simulink model "stackedRotor_dualEMRAX_dynInflow"  (R2022b)
settings: Solver=ode45  StartTime=0.0  StopTime=60  RelTol=1e-4  EnableMultiTasking=on
InitFcn:
  | %Hide scope plots
  | HidHandles = get(0,'ShowHiddenHandles');
  | set(0,'ShowHiddenHandles','On');
  | AllScopeHandles = findobj(0,'Type','Figure','Tag','SIMULINK_SIMSCOPE_FIGURE');
  | close(AllScopeHandles);
  | set(0,'ShowHiddenHandles',HidHandles);
  | 
  | %Load Cl and Cd from potential flow
  | load('C:\Users\msa2925\Box\Matt Lab Stuff\5th Year\Modeling\Look Up Tables\ClCd-1.mat');
  | 
  | %Load dynamic inflow properties (model and rotor_params)
  | load('C:\Users\msa2925\Box\Matt Lab Stuff\5th Year\Modeling\Look Up Tables\DynInflow-1.mat');
  | 
  | 
  | %Atmospheric Properties
  | rho_air    = 1.225;  % air density in kg/m^3
  | mu         = 1.803e-5; % dynamic viscosity [N-s/m^2]
  | 
  | %Emrax 208 Electrical Properties
  | R          = .0122;  %  resistance, ohms, line-line at room temp
  | L          = 125*10^-6;  %  inductance line-line at commutation frequency, henries
  | t_elec     = L/R;
  | Imotor     = 256/100^2;  %  kg*m^2 -- From Emrax data sheet
  | Kt_motor   = .80;  %  N*m/Arms
  | Ke_motor   = .0487*sqrt(2)*60/(2*pi);  %  Vpk/rad/sec
  | Ke         = .0487*sqrt(2)*60/(2*pi);   %radians/sec
  | POLES      = 20;
  | 
  | % no-load current fit (i0 = a1*omega^2 + a2) [Apk]
  | i_a1 = 8.98e-5;
  | i_a2 = 2.51;
  | 
  | %-----------Controller Properties------------------%
  | Vbus                 = 175;  % Actual bus voltage (volts) that will be applied
  | CurrentSenseMax      = 250;  %  Max current sense from controller code
  | BASE_CURRENT         = 125;   %  Max current in amps corresponding to normalized control loop current = 1
  | LOOP_FREQUENCY       = 35;     % orig: 35 in kHz
  | T_LOOP               = .001/LOOP_FREQUENCY;
  | pwm_loop_prescalar   = 1;  %Presacalar how many PWM cycles for one current loop execution
  | T_PWM                = T_LOOP/pwm_loop_prescalar;  %  Current loop prescaler on PWM is 1 for Uber
  | BASE_FREQ            = 1200; %POLES/2*1300/60;  %  1300 rpm
  | BaseSpeed            = BASE_FREQ*(60.0/(POLES/2.0));
  | omega                = 0;               % omega for de-coupling integrator
  | MsgFreq              = 1000; %Hz
  | 
  | %Current loop
  | alpha    = 250*2*pi;         % current loop bandwidth
  | I_Kp     = alpha*L*1;
  | I_Ki     = alpha*R/I_Kp*T_LOOP;
  | 
  | %Speed loop
  | SpeedLoopPrescale  = 5;
  | Tspeedloop         = T_LOOP*SpeedLoopPrescale;
  | PID_spd_Kp         = 4.75;   % From Uber code (ORIGINIAL: 3)
  | % PID_spd_Ki         = 2.1*Tspeedloop*1.5;   % From Uber code (ORIGINAL: 0.15*Tspeedloop*2)
  | PID_spd_Ki         = 1.75*Tspeedloop;
  | 
  | %Position loop
  | speedErrorPEngage    = .003; % Speed error max for position loop to enable
  | % Code has .001 for PEngage, trying something diff here
  | PID_pos_Kp           = 4.75; %on MC40: 2.5 (changed on 23 OCT 2021 to 3.5)
  | PID_pos_Ki           = 1e-3; % orig: 0.00003. increase for faster response.
  | PID_pos_Kd           = 8000; % on MC40: 8000.
  | 
  | PID_pos_error_sat   = .3;  % ORIG = 0.3 Maximum error saturated into position PID (in simulink, not C right now)
  | PID_pos_sat         = 1;  %  From code, based on DC bus limit (orig: .25)
  | PID_pos_C1          = .999; % ORIG = 1 Position loop D bandlimit filter
  | PID_pos_C2          = .001;  % ORIG = 0 Position loop D bandlimit filter
  | 
  | 
  | %transfer function of speed estimator is K1*K3*z/(z-K2)
  | %  Pole is at z = K2
  | % z = exp(-sT)
  | f_estpole = 35000;  %orig: 35000
  | K1        = 1/(BASE_FREQ*T_LOOP);   %  Divide by base freq to convert from elec delta-normalized-angle/cycle to [0,1] normalized speed
  |                                     %  K1 converts delta angle estimate over a loop period to a [0,1] speed estimate
  | K2        = exp(-f_estpole*2*pi*T_LOOP);
  | K3        = 1 - K2;  % Set to make filter have unity gain at 0 frequency (z = 1)
  | 
  | %----------------Rotor properties----------------%
  | d_prop      = 2.216;   %  diameter propeller [m] 2.032 (coax) 2.216 (uber)
  | c           = 0.08; %chord [m]
  | nb          = 2; %number of blades
  | sigma       = nb*c/pi/(d_prop/2);
  | GR          = 1; %gear ratio
  | %Iload        = 0.3578*(1/GR)^2; (coax rotor inertia)
  | %inertias (stacked) measured from 230929 and 231003 testing
  | Im_upper    = 0.3662; %kg-m2
  | Im_lower    = 0.3540;
  | Ir_upper    = 0.3124;
  | Ir_lower    = 0.3317;
  | 
  | %from stacked dual motor testing, coax hubs (220403_test_b)
  | %Iload       = 0.3578/2*(1/GR)^2; %from stacked dual motor testing (231023_test_b)
  | % Iload       = I_eff + Idrive + Imotor;
  | 
  | 
  | %------------Inputs---------------%
  | Ang_slew       = 15.83; % deg/s
  | Ramp_sec       = 100; % rpm/s
  | InitialRPM     = 950*GR;
  | omegamech      = InitialRPM/60*2*pi;  %  Used to preload Q current voltage integrator
  | t_ang_step     = 2; %timestep for angle commands
  | t_swept        = 10; %time to send swept sine input
values from neighbouring files (symbols this model uses):
  AoA_sweep = [-2 -1 0 1 2 3 4 5 6 7 8 9 ... (13 elements, 1x13)]    [ClCd-1.mat]
  Cdl = [0.0123 0.0123 0.0123 0.0123 0.0123 0.0123 0.0123 0.0123 0.0123 0.0123 0.0123 0.0123 ... (6500 elements, 13x500)]    [ClCd-1.mat]
  Cdu = [0.0123 0.0123 0.0123 0.0123 0.0123 0.0123 0.0123 0.0123 0.0123 0.0123 0.0123 0.0123 ... (6500 elements, 13x500)]    [ClCd-1.mat]
  Cll = [-0.111113403346 0.00796289645531 0.127036770682 0.246071948277 0.365032169973 0.483881199334 0.602582833794 0.721100915686 0.839399343253 0.957442081649 1.07519317391 1.19261675192 ... (6500 elements, 13x500)]    [ClCd-1.mat]
  Clu = [-0.11705321178 0.00839337636768 0.133837407812 0.259240671085 0.384564967138 0.509772120977 0.634823993289 0.759682492064 0.884309584192 1.00866730705 1.13271778008 1.2564232163 ... (6500 elements, 13x500)]    [ClCd-1.mat]
  Cp = [0.000195201118563 0.000195344815163 0.000195970524669 0.000196911243155 0.000198292722473 0.000199793715635 0.000201836164013 0.000204359459521 0.00020706119236 0.00020992934584 0.000212955219574 0.000216131124695 ... (150 elements, 1x150)]    [BEMT-1.mat]    (also in BEMT-2.mat = [5.908e-05 5.908e-05 5.908e-05 5.908e-05 5.908e-05 5.908e-05; BEMT-3.mat = [6.167e-05 6.167e-05 6.167e-05 6.167e-05 6.167e-05 6.1671725; BEMT-PF-Isolated-1.mat = [6.88284627296e-05 6.76929537705e-05 6.92283244838e-05 7.518; BEMT-PF-Isolated-2.mat = [6.88286203447e-05 6.76929720507e-05 6.92293837373e-05 7.518)
  Cpl = [0.000333700998998 0.000390181039031 0.000394788670278 0.000400729506228 0.000408611755119 0.000419410254194 0.000434611180529 0.000454621522012 0.000471293145772 0.000468819202162 0.000461044856051 0.0004465872684 ... (37 elements, 1x37)]    [BEMT-PF-Stacked-1.mat]    (also in BEMT-PF-Stacked-3.mat = [0.00012095698162 0.000162284223538 0.000164817714818 0.0001; BEMT-PF-Stacked-4.mat = [0.000215313097577 0.00022323140747 0.000225181363314 0.0002; BEMT-PF-Stacked-5.mat = [0.000201399004141 0.000209364989981 0.000211223578331 0.000; CpData-Stacked-1.mat = [0.0004204989393 0.000429722690454 0.000432518606247 0.00043)
  Cpu = [0.000372640330495 0.000318761476241 0.00031503993434 0.000310316169544 0.000304143730405 0.000295773643033 0.00028387117424 0.000265492168428 0.000237641915024 0.000230728320611 0.000223594040333 0.000216887343718 ... (37 elements, 1x37)]    [BEMT-PF-Stacked-1.mat]    (also in BEMT-PF-Stacked-3.mat = [0.00014995136179 0.000108984048023 0.00010569458686 0.00010; BEMT-PF-Stacked-4.mat = [0.000200079302516 0.0001931098957 0.000191441123461 0.00018; BEMT-PF-Stacked-5.mat = [0.000223261524278 0.000214635121691 0.000212581398187 0.000; CpData-Stacked-1.mat = [0.000470292570894 0.000463315827435 0.000462372188797 0.000)
  Ct = [0 8.42066058624e-05 0.000168413211725 0.000252619817587 0.000348569118235 0.000435711397794 0.000522853677352 0.000609995956911 0.00069713823647 0.000784280516029 0.000871422795587 0.000958565075146 ... (150 elements, 1x150)]    [BEMT-1.mat]    (also in BEMT-2.mat = [-0.000241284312952 -0.00019885713846 -0.000156429963968 -0.; BEMT-3.mat = [-0.000252881464423 -0.00020500571035 -0.00015767832519 -0.0; BEMT-PF-Isolated-1.mat = [-0.000124730397385 6.78902114512e-07 0.000152796242494 0.00; BEMT-PF-Isolated-2.mat = [-0.000124743531158 6.68801957239e-07 0.000152879013625 0.00)
  Ctl = [0.00438668608339 0.0050628698524 0.00511522584539 0.00518172746808 0.00526807639226 0.00538256546486 0.00553531477508 0.00571551109899 0.00580582681419 0.00575766596858 0.00565748394784 0.00549586936617 ... (37 elements, 1x37)]    [BEMT-PF-Stacked-1.mat]    (also in BEMT-PF-Stacked-2.mat = [0.00446656952376 0.00504151525843 0.00508284852112 0.005134; BEMT-PF-Stacked-3.mat = [0.00184996435909 0.00209589101081 0.00210506301257 0.002127; BEMT-PF-Stacked-4.mat = [0.00305779502317 0.00317485141984 0.00320289061972 0.003237; BEMT-PF-Stacked-5.mat = [0.00284078729023 0.00295761000687 0.00298453442892 0.003017)
  Ctu = [0.00485875244254 0.00420098979139 0.00415434112966 0.00409491081367 0.00401692201007 0.00391066006909 0.00375881977479 0.00352379292731 0.0031675839941 0.00307949239151 0.00298865074931 0.00290335167779 ... (37 elements, 1x37)]    [BEMT-PF-Stacked-1.mat]    (also in BEMT-PF-Stacked-2.mat = [0.00487929290239 0.00430977798758 0.00426987840094 0.004219; BEMT-PF-Stacked-3.mat = [0.00202552929257 0.00178155832272 0.00175724958711 0.001735; BEMT-PF-Stacked-4.mat = [0.00282403441036 0.00271496837402 0.00268870985611 0.002655; BEMT-PF-Stacked-5.mat = [0.00315608603824 0.00303364263049 0.00300412792098 0.002966)
  index_sweep = [-90 -45 -40 -35 -30 -25 -20 -15 -10 -9 -8 -7 ... (37 elements, 1x37)]    [BEMT-PF-Stacked-1.mat]    (also in BEMT-PF-Stacked-2.mat; BEMT-PF-Stacked-3.mat = [-90 -45 -40 -35 -30 -25 -20 -15 -14 -13 -12 -11 ... (45 ele; BEMT-PF-Stacked-4.mat; BEMT-PF-Stacked-5.mat)
  index_sweep_Cp_table = [-90 -45.2679945682 -41.0748847617 -35.9788199136 -30.8261561384 -25.6873115637 -20.5477936424 -15.3629851439 -10.3005197032 -7.23856497031 -5.29357093665 -4.47027434572 ... (27 elements, 1x27)]    [CpData-Stacked-1.mat]
  model =     [DynInflow-1.mat]    (also in PP-1.mat; PP-2.mat; PP-3.mat)
  rotor_params =     [DynInflow-1.mat]    (also in PP-1.mat; PP-2.mat; PP-3.mat)
  theta = [-1.24244156171 -0.730247869575 -0.489791195362 -0.291308360013 -0.0904887039498 0.0775201787218 0.236938510902 0.389966557012 0.537998944025 0.680941129328 0.820002111662 0.955737387113 ... (150 elements, 1x150)]    [BEMT-1.mat]    (also in BEMT-2.mat = [-2.67472972391 -2.52181622329 -2.35655527709 -2.17339529035; BEMT-3.mat = [-2.61565298703 -2.45920727031 -2.29202818901 -2.11251263407; BEMT-PF-Isolated-1.mat = [-2 -1 0 1 2 3 4 5 6 7 8 9 ... (16 elements, 1x16)]; BEMT-PF-Isolated-2.mat = [-2 -1 0 1 2 3 4 5 6 7 8 9 ... (16 elements, 1x16)])
  x_sweep = [-1.74044233009 -1.73346660933 -1.72649088856 -1.7195151678 -1.71253944704 -1.70556372628 -1.69858800552 -1.69161228476 -1.68463656399 -1.67766084323 -1.67068512247 -1.66370940171 ... (500 elements, 1x500)]    [ClCd-1.mat]
undefined symbols (not defined in the file or in its folder): DiscIntNeverNeededParam
libraries: dspsrcs4 x2
(part 1 of 2)
settings Model: ModifiedHistory=4/7/2020 Adding in voltage saturation to mag 1 before SVGEN  Creator=mricci  LastModifiedBy=msa2925
settings SolverCC: AlgebraicLoopSolver=TrustRegion
settings DataIOCC: LimitDataPoints=on  SaveFormat=Array  SignalLoggingSaveFormat=ModelDataLogs  ReturnWorkspaceOutputs=off
settings OptimizationCC: ReuseModelBlockBuffer=on  ExpressionDepthLimit=2147483647  InitFltsAndDblsToZero=on  LifeSpan=inf
settings DebuggingCC: UnderspecifiedInitializationDetection=Classic  MergeDetectMultiDrivingBlocksExec=none  SolverPrmCheckMsg=warning  FcnCallInpInsideContextMsg=warning  UnconnectedInputMsg=warning  UnconnectedOutputMsg=warning  UnconnectedLineMsg=warning  StateNameClashWarn=warning  SFUnexpectedBacktrackingDiag=warning  SFNoUnconditionalDefaultTransitionDiag=warning  SFExecutionAtInitializationDiag=none  ArithmeticOperatorsInVariantConditions=warning
settings HardwareCC: ProdBitPerPointer=32  ProdBitPerSizeT=32  ProdBitPerPtrDiffT=32  ProdLargestAtomicFloat=None  ProdIntDivRoundTo=Undefined  ProdEndianess=Unspecified  ProdWordSize=32  ProdHWDeviceType=32-bit Generic
settings ModelReferenceCC: EnableRefExpFcnMdlSchedulingChecks=on  PropagateSignalLabelsOutOfModel=off
settings RTWCC: DLArmComputeVersion=19.05
settings CodeAppCC: StateflowObjectComments=on
settings GRTTargetCC: TargetLangStandard=C89/C90 (ANSI)  CombineOutputUpdateFcns=off  GRTInterface=on
settings ConfigComp: CovMetricSettings=dw  CovSaveCumulativeToWorkspaceVar=on  CovSaveSingleToWorkspaceVar=on

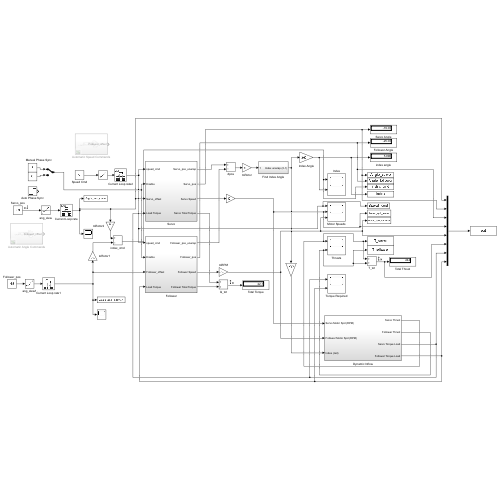
[thumbnail: Simulink's stored preview of the top-level diagram]
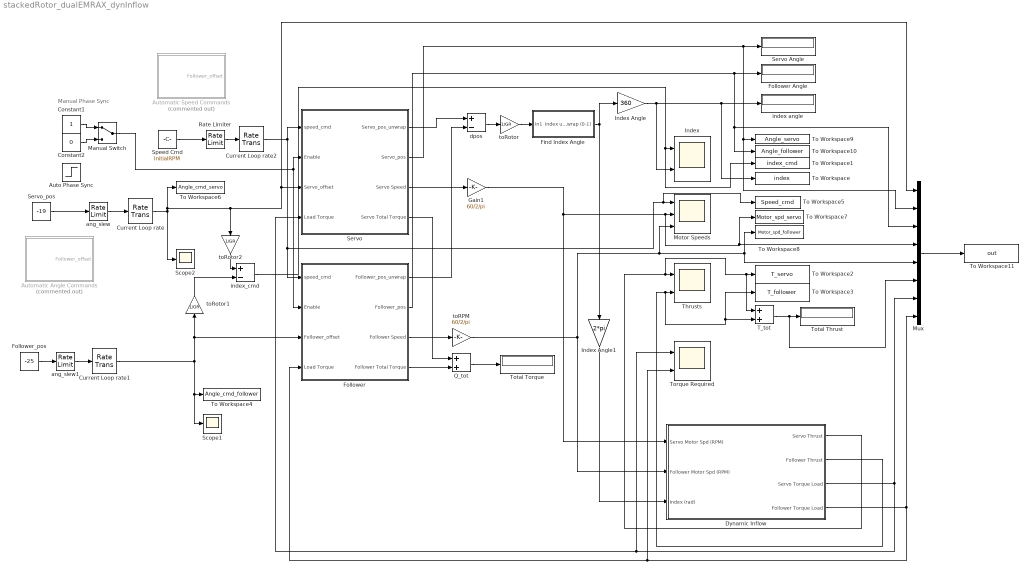
== system stackedRotor_dualEMRAX_dynInflow ==
  note: Manual Phase Sync
  Auto Phase Sync : Step  Time=3  SampleTime=0
  Automatic Angle Commands : Subsystem  Commented=on
  Automatic Speed Commands : Subsystem  Commented=on
  Constant1 : Constant
  Constant2 : Constant  Value=0
  Current Loop rate : RateTransition  OutPortSampleTime=T_LOOP
  Current Loop rate1 : RateTransition  OutPortSampleTime=T_LOOP
  Current Loop rate2 : RateTransition  OutPortSampleTime=T_LOOP
  Dynamic Inflow : Subsystem
  Find Index Angle : Subsystem
  Follower : Subsystem
  Follower Angle : Display
  Follower_pos : Constant  Value=-25
  Gain1 : Gain  Gain=60/2/pi
  Index : Scope  NumInputPorts=2
  Index Angle : Gain  Gain=360
  Index Angle1 : Gain  Gain=2*pi
  Manual Switch : ManualSwitch
  Motor Speeds : Scope  NumInputPorts=3
  Mux : Mux  Inputs=8
  Q_tot : Sum
  Rate Limiter : RateLimiter  RisingSlewLimit=Ramp_sec  FallingSlewLimit=-Ramp_sec  SampleTimeMode=inherited  InitialCondition=InitialRPM/BaseSpeed
  Scope1 : Scope
  Scope2 : Scope
  Servo : Subsystem
  Servo Angle : Display
  Servo_pos : Constant  Value=-19
  Speed Cmd : Constant  Value=InitialRPM
  T_tot : Sum
  Thrusts : Scope  NumInputPorts=2
  To Workspace : ToWorkspace  VariableName=index  SaveFormat=Timeseries  SampleTime=-1
  To Workspace1 : ToWorkspace  VariableName=index_cmd  SaveFormat=Timeseries  SampleTime=-1
  To Workspace10 : ToWorkspace  VariableName=Angle_follower  SaveFormat=Timeseries  SampleTime=-1
  To Workspace11 : ToWorkspace  VariableName=out  SaveFormat=Timeseries  SampleTime=-1
  To Workspace2 : ToWorkspace  VariableName=T_servo  SaveFormat=Timeseries  SampleTime=-1
  To Workspace3 : ToWorkspace  VariableName=T_follower  SaveFormat=Timeseries  SampleTime=-1
  To Workspace4 : ToWorkspace  VariableName=Angle_cmd_follower  SaveFormat=Timeseries  SampleTime=-1
  To Workspace5 : ToWorkspace  VariableName=Speed_cmd  SaveFormat=Timeseries  SampleTime=-1
  To Workspace6 : ToWorkspace  VariableName=Angle_cmd_servo  SaveFormat=Timeseries  SampleTime=-1
  To Workspace7 : ToWorkspace  VariableName=Motor_spd_servo  SaveFormat=Timeseries  SampleTime=-1
  To Workspace8 : ToWorkspace  VariableName=Motor_spd_follower  SaveFormat=Timeseries  SampleTime=-1
  To Workspace9 : ToWorkspace  VariableName=Angle_servo  SaveFormat=Timeseries  SampleTime=-1
  Torque Required : Scope  NumInputPorts=2
  Total Thrust : Display
  Total Torque : Display
  ang_slew : RateLimiter  RisingSlewLimit=Ang_slew  FallingSlewLimit=-Ang_slew  SampleTimeMode=inherited
  ang_slew1 : RateLimiter  RisingSlewLimit=Ang_slew  FallingSlewLimit=-Ang_slew  SampleTimeMode=inherited
  dpos : Sum  Inputs=+-
  index angle : Display
  index_cmd : Sum  Inputs=+-
  toRPM : Gain  Gain=60/2/pi
  toRotor : Gain  Gain=1/GR
  toRotor1 : Gain  Gain=1/GR
  toRotor2 : Gain  Gain=1/GR
  wires:
  Speed Cmd/1 -> Rate Limiter/1
  toRPM/1 -> Motor Speeds/3, Mux/5, To Workspace8/1, Dynamic Inflow/2(Follower Motor Spd (RPM))
  Current Loop rate2/1 -> Servo/1(speed_cmd), Follower/1(speed_cmd), Motor Speeds/1, To Workspace5/1
  Servo/3(Servo Speed) -> Gain1/1
  Current Loop rate/1 -> To Workspace6/1, Mux/1, Servo/3(Servo_offset), toRotor2/1, Scope2/1
  Servo/1(Servo_pos_unwrap) -> dpos/1
  index_cmd/1 -> To Workspace1/1, Index/1
  Index Angle/1 -> index angle/1, To Workspace/1, Index/2
  dpos/1 -> toRotor/1
  toRotor/1 -> Find Index Angle/1(In1)
  Find Index Angle/1(Index unwrap (0-1)) -> Index Angle1/1, Index Angle/1
  Servo/2(Servo_pos) -> To Workspace9/1, Mux/2, Servo Angle/1
  Dynamic Inflow/1(Servo Thrust) -> T_tot/1, To Workspace2/1, Thrusts/1
  Dynamic Inflow/3(Servo Torque Load) -> Mux/7, Torque Required/1, Servo/4(Load Torque)
  Follower/1(Follower_pos_unwrap) -> dpos/2
  Follower/3(Follower Speed) -> toRPM/1
  Follower/2(Follower_pos) -> Follower Angle/1, To Workspace10/1, Mux/3
  T_tot/1 -> Mux/6, Total Thrust/1
  Rate Limiter/1 -> Current Loop rate2/1
  ang_slew/1 -> Current Loop rate/1
  toRotor2/1 -> index_cmd/1
  toRotor1/1 -> index_cmd/2
  Manual Switch/1 -> Follower/2(Enable), Servo/2(Enable)
  Current Loop rate1/1 -> toRotor1/1, Follower/3(Follower_offset), Scope1/1, To Workspace4/1
  Mux/1 -> To Workspace11/1
  Constant1/1 -> Manual Switch/1
  Constant2/1 -> Manual Switch/2
  Follower_pos/1 -> ang_slew1/1
  ang_slew1/1 -> Current Loop rate1/1
  Follower/4(Follower Total Torque) -> Q_tot/2
  Servo/4(Servo Total Torque) -> Q_tot/1
  Q_tot/1 -> Total Torque/1
  Servo_pos/1 -> ang_slew/1
  Gain1/1 -> Dynamic Inflow/1(Servo Motor Spd (RPM)), Motor Speeds/2, To Workspace7/1, Mux/4
  Dynamic Inflow/4(Follower Torque Load) -> Torque Required/2, Follower/4(Load Torque), Mux/8
  Dynamic Inflow/2(Follower Thrust) -> T_tot/2, To Workspace3/1, Thrusts/2
  Index Angle1/1 -> Dynamic Inflow/3(Index (rad))

== system stackedRotor_dualEMRAX_dynInflow/Automatic Angle Commands ==
  Ang_cmds : Constant  Value=[-151 -151 -151 -147.7 -147.7 -147.7 -147.7 -147.7]  VectorParams1D=off
  Clock : Clock
  Current Loop rate : RateTransition  OutPortSampleTime=T_LOOP
  Enabled Subsystem : Subsystem  TreatAsAtomicUnit=on
  Enabled Subsystem1 : Subsystem  TreatAsAtomicUnit=on
  Floor : Rounding
  Follower_pos : Selector  IndexMode=Zero-based  InputPortWidth=8  IndexOptions=Index vector (port)  Indices=[1 3]  OutputSizes=1
  Gain : Gain  Gain=1/t_ang_step
  GreaterThanOrEqual : RelationalOperator  OutDataTypeStr=boolean  RndMeth=Simplest  InputSameDT=off
  Merge1 : Merge
  NOT : Logic  Operator=NOT  IconShape=distinctive  AllPortsSameDT=off  OutDataTypeStr=boolean
  Time to swept sine : Constant  Value=t_swept/t_ang_step
  ang_slew1 : RateLimiter  RisingSlewLimit=Ang_slew  FallingSlewLimit=-Ang_slew  SampleTimeMode=inherited
  Follower_offset : Outport
  wires:
  Floor/1 -> GreaterThanOrEqual/1, Follower_pos/2
  Gain/1 -> Floor/1
  Enabled Subsystem1/1(Out1) -> Merge1/2
  GreaterThanOrEqual/1 -> Enabled Subsystem/Enable, NOT/1
  Time to swept sine/1 -> GreaterThanOrEqual/2
  NOT/1 -> Enabled Subsystem1/Enable
  Follower_pos/1 -> ang_slew1/1
  Clock/1 -> Gain/1
  Current Loop rate/1 -> Enabled Subsystem/1(In1), Enabled Subsystem1/1(In1)
  Ang_cmds/1 -> Follower_pos/1
  Enabled Subsystem/1(Out1) -> Merge1/1
  ang_slew1/1 -> Current Loop rate/1
  Merge1/1 -> Follower_offset/1

== system stackedRotor_dualEMRAX_dynInflow/Automatic Speed Commands ==
  Ang_cmds : Constant  Value=ones(1,8)*InitialRPM
  Clock : Clock
  Current Loop rate : RateTransition  OutPortSampleTime=T_LOOP
  Enabled Subsystem : Subsystem  TreatAsAtomicUnit=on
  Enabled Subsystem1 : Subsystem  TreatAsAtomicUnit=on
  Floor : Rounding
  Follower_pos : Selector  IndexMode=Zero-based  InputPortWidth=8  IndexOptions=Index vector (port)  Indices=[1 3]  OutputSizes=1
  Gain : Gain  Gain=1/t_ang_step
  GreaterThanOrEqual : RelationalOperator  OutDataTypeStr=boolean  RndMeth=Simplest  InputSameDT=off
  Merge1 : Merge
  NOT : Logic  Operator=NOT  IconShape=distinctive  AllPortsSameDT=off  OutDataTypeStr=boolean
  Time to swept sine : Constant  Value=t_swept/t_ang_step
  ang_slew1 : RateLimiter  RisingSlewLimit=Ramp_sec  FallingSlewLimit=-Ramp_sec  SampleTimeMode=inherited
  Follower_offset : Outport
  wires:
  Floor/1 -> GreaterThanOrEqual/1, Follower_pos/2
  Gain/1 -> Floor/1
  Enabled Subsystem1/1(Out1) -> Merge1/2
  GreaterThanOrEqual/1 -> Enabled Subsystem/Enable, NOT/1
  Time to swept sine/1 -> GreaterThanOrEqual/2
  NOT/1 -> Enabled Subsystem1/Enable
  Follower_pos/1 -> ang_slew1/1
  Clock/1 -> Gain/1
  Current Loop rate/1 -> Enabled Subsystem/1(In1), Enabled Subsystem1/1(In1)
  Ang_cmds/1 -> Follower_pos/1
  Enabled Subsystem/1(Out1) -> Merge1/1
  ang_slew1/1 -> Current Loop rate/1
  Merge1/1 -> Follower_offset/1

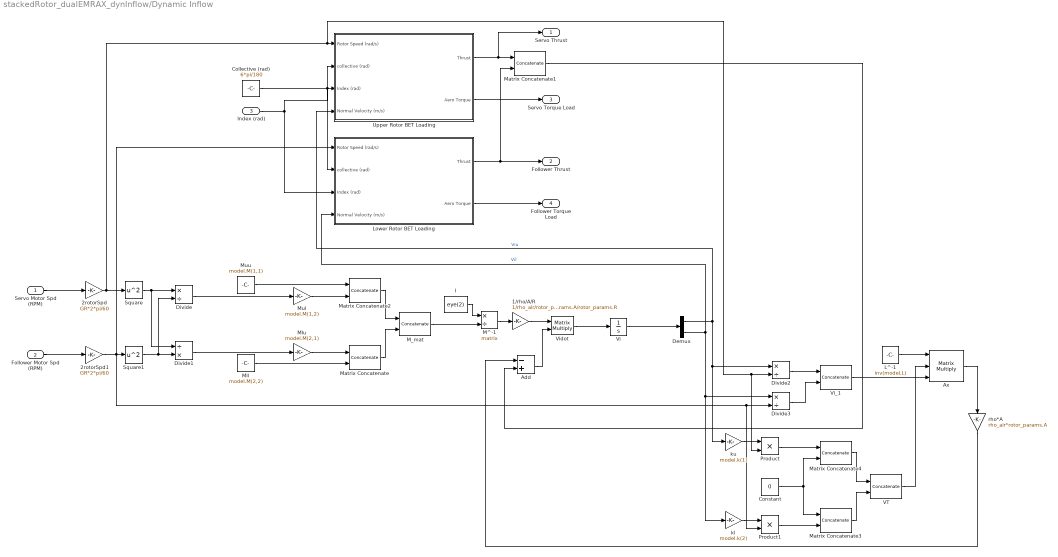
== system stackedRotor_dualEMRAX_dynInflow/Dynamic Inflow ==
  Servo Motor Spd (RPM) : Inport
  Follower Motor Spd (RPM) : Inport  Port=2
  Index (rad) : Inport  Port=3
  1/rho/A/R : Gain  Gain=1/rho_air/rotor_params.A/rotor_params.R
  2rotorSpd : Gain  Gain=GR*2*pi/60
  2rotorSpd1 : Gain  Gain=GR*2*pi/60
  Add : Sum  Inputs=-+
  Ax : Product  Inputs=3  Multiplication=Matrix(*)  RndMeth=Zero
  Collective (rad) : Constant  Value=6*pi/180
  Constant : Constant  Value=0
  Demux : Demux  Outputs=2
  Divide : Product  Inputs=*/
  Divide1 : Product  Inputs=/*
  Divide2 : Product  Inputs=*/
  Divide3 : Product  Inputs=*/
  I : Constant  Value=eye(2)
  L^-1 : Constant  Value=inv(model.L)
  Lower Rotor BET Loading : Subsystem
  M^-1 : Product  Inputs=*/  Multiplication=Matrix(*)
  M_mat : Concatenate  Mode=Multidimensional array
  Matrix Concatenate{,1..4} (5 alike) : Concatenate  Mode=Multidimensional array  ConcatenateDimension=2
  Mll : Constant  Value=model.M(2,2)
  Mlu : Gain  Gain=model.M(2,1)
  Mul : Gain  Gain=model.M(1,2)
  Muu : Constant  Value=model.M(1,1)
  Product : Product
  Product1 : Product
  Square : Math  Operator=square
  Square1 : Math  Operator=square
  Upper Rotor BET Loading : Subsystem
  VT : Concatenate  Mode=Multidimensional array
  Vi : Integrator  InitialCondition=[5;7]
  Vi_1 : Concatenate  Mode=Multidimensional array
  Vidot : Product  Multiplication=Matrix(*)  RndMeth=Zero
  kl : Gain  Gain=model.k(2)
  ku : Gain  Gain=model.k(1)
  rho*A : Gain  Gain=rho_air*rotor_params.A
  Servo Thrust : Outport
  Follower Thrust : Outport  Port=2
  Servo Torque Load : Outport  Port=3
  Follower Torque Load : Outport  Port=4
  wires:
  2rotorSpd/1 -> Square/1, Product/2, Divide2/2, Upper Rotor BET Loading/1(Rotor Speed (rad/s))
  Demux/1 -> Upper Rotor BET Loading/4(Normal Velocity (m/s)), ku/1, Divide2/1  "Viu"
  Matrix Concatenate3/1 -> VT/2
  Matrix Concatenate/1 -> M_mat/2
  1/rho/A/R/1 -> Vidot/1
  L^-1/1 -> Ax/1
  Divide1/1 -> Mlu/1
  2rotorSpd1/1 -> Lower Rotor BET Loading/1(Rotor Speed (rad/s)), Divide3/2, Product1/2, Square1/1
  Square1/1 -> Divide1/2, Divide/2
  Matrix Concatenate1/1 -> Add/2
  Constant/1 -> Matrix Concatenate4/2, Matrix Concatenate3/1
  ku/1 -> Product/1
  Demux/2 -> Lower Rotor BET Loading/4(Normal Velocity (m/s)), Divide3/1, kl/1  "Vil"
  Muu/1 -> Matrix Concatenate2/1
  Lower Rotor BET Loading/1(Thrust) -> Follower Thrust/1, Matrix Concatenate1/2
  Vi/1 -> Demux/1
  Upper Rotor BET Loading/1(Thrust) -> Matrix Concatenate1/1, Servo Thrust/1
  Divide/1 -> Mul/1
  Ax/1 -> rho*A/1
  Vi_1/1 -> Ax/3
  Mll/1 -> Matrix Concatenate/2
  Follower Motor Spd (RPM)/1 -> 2rotorSpd1/1
  Product1/1 -> Matrix Concatenate3/2
  M_mat/1 -> M^-1/2
  kl/1 -> Product1/1
  Matrix Concatenate2/1 -> M_mat/1
  Add/1 -> Vidot/2
  Collective (rad)/1 -> Lower Rotor BET Loading/2(collective (rad)), Upper Rotor BET Loading/2(collective (rad))
  VT/1 -> Ax/2
  Product/1 -> Matrix Concatenate4/1
  Mul/1 -> Matrix Concatenate2/2
  Divide3/1 -> Vi_1/2
  Servo Motor Spd (RPM)/1 -> 2rotorSpd/1
  Square/1 -> Divide1/1, Divide/1
  Mlu/1 -> Matrix Concatenate/1
  Lower Rotor BET Loading/2(Aero Torque) -> Follower Torque Load/1
  Divide2/1 -> Vi_1/1
  I/1 -> M^-1/1
  M^-1/1 -> 1/rho/A/R/1
  Matrix Concatenate4/1 -> VT/1
  Vidot/1 -> Vi/1
  Upper Rotor BET Loading/2(Aero Torque) -> Servo Torque Load/1
  Index (rad)/1 -> Lower Rotor BET Loading/3(Index (rad)), Upper Rotor BET Loading/3(Index (rad))
  rho*A/1 -> Add/1

== system stackedRotor_dualEMRAX_dynInflow/Find Index Angle ==
  In1 : Inport
  If : If  IfExpression=u1 >= 0
  If Action Subsystem : Subsystem  TreatAsAtomicUnit=on
  If Action Subsystem1 : Subsystem  TreatAsAtomicUnit=on
  If Action Subsystem2 : Subsystem  TreatAsAtomicUnit=on
  If Action Subsystem3 : Subsystem  TreatAsAtomicUnit=on
  If Action Subsystem4 : Subsystem  TreatAsAtomicUnit=on
  If1 : If  IfExpression=".25 < u1  & u1 <= .75"  ElseIfExpressions=u1 > .75
  Merge : Merge
  Merge1 : Merge  Inputs=3
  Product : Product
  Sign : Signum
  Index unwrap (0-1) : Outport
  wires:
  In1/1 -> If Action Subsystem/1(In1), Sign/1, If Action Subsystem1/1(In1), If/1
  If/1 -> If Action Subsystem/Action
  If/2 -> If Action Subsystem1/Action
  If Action Subsystem/1(Out1) -> Merge/1
  If Action Subsystem1/1(Out1) -> Merge/2
  Merge/1 -> If Action Subsystem3/1(In1), If Action Subsystem4/1(In1), If Action Subsystem2/1(In1), If1/1
  If1/1 -> If Action Subsystem2/Action
  If1/2 -> If Action Subsystem3/Action
  If1/3 -> If Action Subsystem4/Action
  If Action Subsystem3/1(Out1) -> Merge1/2
  If Action Subsystem2/1(Out1) -> Merge1/1
  If Action Subsystem4/1(Out1) -> Merge1/3
  Merge1/1 -> Product/2
  Sign/1 -> Product/1
  Product/1 -> Index unwrap (0-1)/1

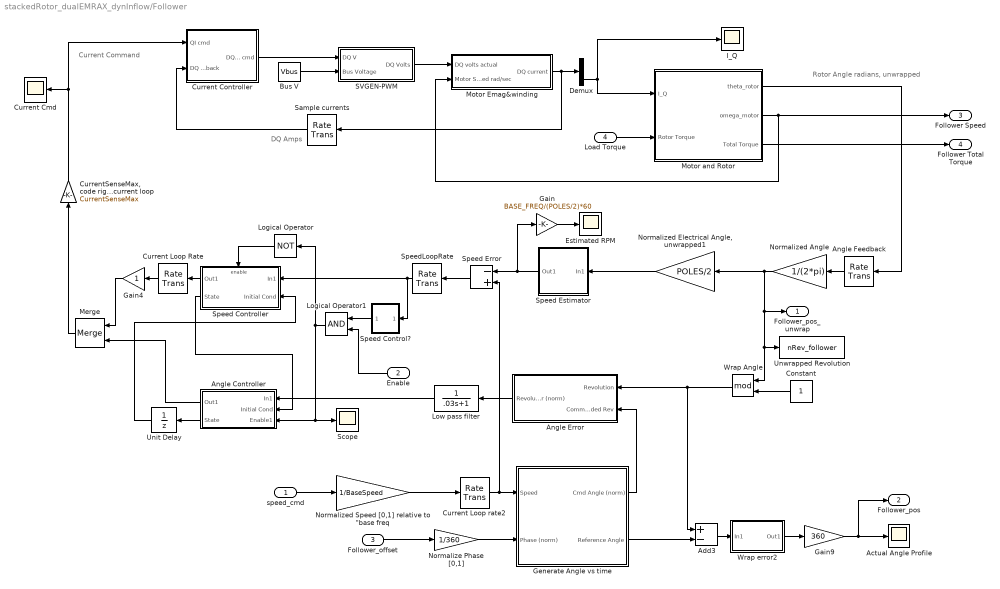
== system stackedRotor_dualEMRAX_dynInflow/Follower ==
  note: Current Command
  note: Rotor Angle radians, unwrapped
  note: DQ Amps
  speed_cmd : Inport
  Enable : Inport  Port=2
  Follower_offset : Inport  Port=3
  Load Torque : Inport  Port=4
  Actual Angle Profile : Scope
  Add3 : Sum  Inputs=+-
  Angle Controller : Subsystem  TreatAsAtomicUnit=on
  Angle Error : Subsystem
  Angle Feedback : RateTransition  OutPortSampleTime=T_LOOP
  Bus V : Constant  Value=Vbus
  Constant : Constant
  Current Loop Rate : RateTransition  OutPortSampleTime=T_LOOP
  Current Cmd : Scope
  Current Controller : Subsystem
  Current Loop rate2 : RateTransition  OutPortSampleTime=T_LOOP
  "CurrentSenseMax, code right now has Controller outputting PU amps then scaled to amps going into current loop" : Gain  Gain=CurrentSenseMax
  Demux : Demux  Outputs=2
  Estimated RPM : Scope
  Gain : Gain  Gain=BASE_FREQ/(POLES/2)*60
  Gain4 : Gain
  Gain9 : Gain  Gain=360
  Generate Angle vs time : Subsystem
  I_Q : Scope
  Logical Operator : Logic  Operator=NOT  AllPortsSameDT=off  OutDataTypeStr=boolean
  Logical Operator1 : Logic  AllPortsSameDT=off  OutDataTypeStr=boolean
  Low pass filter : TransferFcn  Denominator=[.03 1]
  Merge : Merge
  Motor Emag&winding : Subsystem
  Motor and Rotor : Subsystem
  Normalize Phase [0,1] : Gain  Gain=1/360
  Normalized Angle : Gain  Gain=1/(2*pi)
  "Normalized Electrical Angle, unwrapped1" : Gain  Gain=POLES/2
  "Normalized Speed [0,1] relative to \"base freq" : Gain  Gain=1/BaseSpeed
  SVGEN-PWM : Subsystem
  Sample currents : RateTransition  OutPortSampleTime=T_LOOP
  Scope : Scope
  Speed Control? : Subsystem
  Speed Controller : Subsystem
  Speed Error : Sum  Inputs=-+
  Speed Estimator : Subsystem
  SpeedLoopRate : RateTransition  OutPortSampleTime=T_LOOP*SpeedLoopPrescale
  Unit Delay : UnitDelay
  Unwrapped Revolution : ToWorkspace  VariableName=nRev_follower  SaveFormat=Timeseries  SampleTime=-1
  Wrap Angle : Math  Operator=mod  SignedPower=on
  Wrap error2 : Subsystem
  Follower_pos_unwrap : Outport
  Follower_pos : Outport  Port=2
  Follower Speed : Outport  Port=3
  Follower Total Torque : Outport  Port=4
  wires:
  speed_cmd/1 -> "Normalized Speed [0,1] relative to \"base freq"/1
  Gain/1 -> Estimated RPM/1
  Speed Control?/1(Out1) -> Logical Operator1/1
  Bus V/1 -> SVGEN-PWM/2(Bus Voltage)
  Enable/1 -> Logical Operator1/2
  Angle Feedback/1 -> Normalized Angle/1
  "Normalized Electrical Angle, unwrapped1"/1 -> Speed Estimator/1(In1)
  Generate Angle vs time/2(Reference Angle) -> Add3/2
  Normalized Angle/1 -> "Normalized Electrical Angle, unwrapped1"/1, Follower_pos_unwrap/1, Unwrapped Revolution/1, Wrap Angle/1
  Constant/1 -> Wrap Angle/2
  Add3/1 -> Wrap error2/1(In1)
  Current Controller/1(DQ V cmd) -> SVGEN-PWM/1(DQ V)
  Motor and Rotor/1(theta_rotor) -> Angle Feedback/1
  Speed Controller/2(State) -> Angle Controller/2(Initial Cond)
  Motor and Rotor/2(omega_motor) -> Follower Speed/1, Motor Emag&winding/2(Motor Speed rad/sec)
  Wrap error2/1(Out1) -> Gain9/1
  Generate Angle vs time/1(Cmd Angle (norm)) -> Angle Error/2(Commanded Rev)
  Gain9/1 -> Follower_pos/1, Actual Angle Profile/1
  Logical Operator/1 -> Speed Controller/Enable
  Speed Error/1 -> SpeedLoopRate/1
  Angle Controller/2(State) -> Unit Delay/1
  Demux/2 -> I_Q/1, Motor and Rotor/1(I_Q)
  Unit Delay/1 -> Speed Controller/2(Initial Cond)
  Logical Operator1/1 -> Angle Controller/3(Enable1), Scope/1, Logical Operator/1
  Speed Estimator/1(Out1) -> Gain/1, Speed Error/1
  Speed Controller/1(Out1) -> Current Loop Rate/1
  "Normalized Speed [0,1] relative to \"base freq"/1 -> Current Loop rate2/1
  Motor Emag&winding/1(DQ current) -> Demux/1, Sample currents/1
  SpeedLoopRate/1 -> Speed Control?/1(In1), Speed Controller/1(In1)
  SVGEN-PWM/1(DQ Volts) -> Motor Emag&winding/1(DQ volts actual)
  Sample currents/1 -> Current Controller/2(DQ I feedback)
  Wrap Angle/1 -> Add3/1, Angle Error/1(Revolution)
  Current Loop rate2/1 -> Speed Error/2, Generate Angle vs time/1(Speed)
  Current Loop Rate/1 -> Gain4/1
  Angle Error/1(Revolution Error (norm)) -> Low pass filter/1
  Low pass filter/1 -> Angle Controller/1(In1)
  "CurrentSenseMax, code right now has Controller outputting PU amps then scaled to amps going into current loop"/1 -> Current Controller/1(QI cmd), Current Cmd/1
  Gain4/1 -> Merge/1
  Merge/1 -> "CurrentSenseMax, code right now has Controller outputting PU amps then scaled to amps going into current loop"/1
  Angle Controller/1(Out1) -> Merge/2
  Follower_offset/1 -> Normalize Phase [0,1]/1
  Normalize Phase [0,1]/1 -> Generate Angle vs time/2(Phase (norm))
  Motor and Rotor/3(Total Torque) -> Follower Total Torque/1
  Load Torque/1 -> Motor and Rotor/2(Rotor Torque)

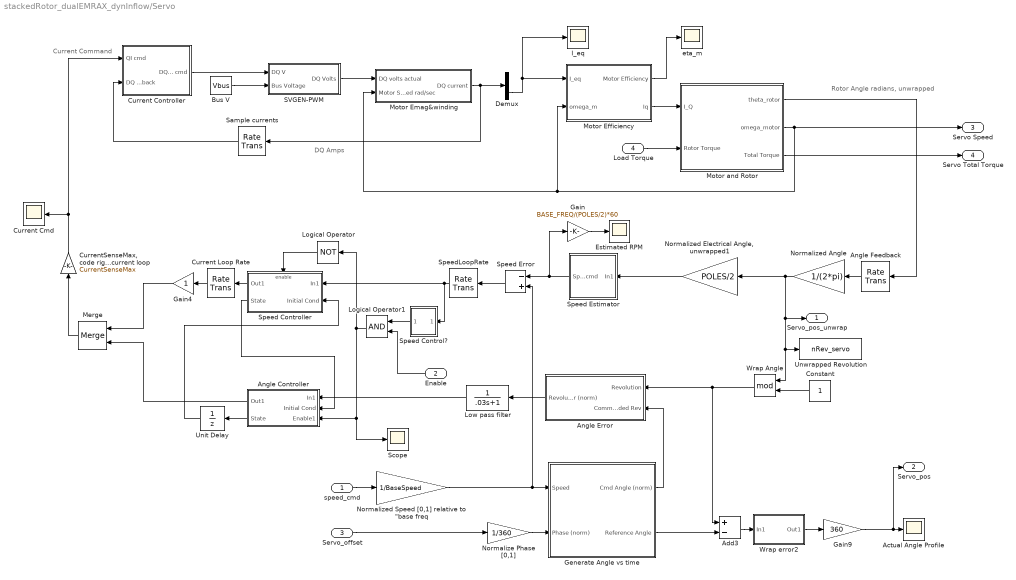
== system stackedRotor_dualEMRAX_dynInflow/Servo ==
  note: Current Command
  note: Rotor Angle radians, unwrapped
  note: DQ Amps
  speed_cmd : Inport
  Enable : Inport  Port=2
  Servo_offset : Inport  Port=3
  Load Torque : Inport  Port=4
  Actual Angle Profile : Scope
  Add3 : Sum  Inputs=+-
  Angle Controller : Subsystem  TreatAsAtomicUnit=on
  Angle Error : Subsystem
  Angle Feedback : RateTransition  OutPortSampleTime=T_LOOP
  Bus V : Constant  Value=Vbus
  Constant : Constant
  Current Loop Rate : RateTransition  OutPortSampleTime=T_LOOP
  Current Cmd : Scope
  Current Controller : Subsystem
  "CurrentSenseMax, code right now has Controller outputting PU amps then scaled to amps going into current loop" : Gain  Gain=CurrentSenseMax
  Demux : Demux  Outputs=2
  Estimated RPM : Scope
  Gain : Gain  Gain=BASE_FREQ/(POLES/2)*60
  Gain4 : Gain
  Gain9 : Gain  Gain=360
  Generate Angle vs time : Subsystem
  I_eq : Scope
  Logical Operator : Logic  Operator=NOT  AllPortsSameDT=off  OutDataTypeStr=boolean
  Logical Operator1 : Logic  AllPortsSameDT=off  OutDataTypeStr=boolean
  Low pass filter : TransferFcn  Denominator=[.03 1]
  Merge : Merge
  Motor Efficiency : Subsystem
  Motor Emag&winding : Subsystem
  Motor and Rotor : Subsystem
  Normalize Phase [0,1] : Gain  Gain=1/360
  Normalized Angle : Gain  Gain=1/(2*pi)
  "Normalized Electrical Angle, unwrapped1" : Gain  Gain=POLES/2
  "Normalized Speed [0,1] relative to \"base freq" : Gain  Gain=1/BaseSpeed
  SVGEN-PWM : Subsystem
  Sample currents : RateTransition  OutPortSampleTime=T_LOOP
  Scope : Scope
  Speed Control? : Subsystem
  Speed Controller : Subsystem
  Speed Error : Sum  Inputs=-+
  Speed Estimator : Subsystem
  SpeedLoopRate : RateTransition  OutPortSampleTime=T_LOOP*SpeedLoopPrescale
  Unit Delay : UnitDelay
  Unwrapped Revolution : ToWorkspace  VariableName=nRev_servo  SaveFormat=Timeseries  SampleTime=-1
  Wrap Angle : Math  Operator=mod  SignedPower=on
  Wrap error2 : Subsystem
  eta_m : Scope
  Servo_pos_unwrap : Outport
  Servo_pos : Outport  Port=2
  Servo Speed : Outport  Port=3
  Servo Total Torque : Outport  Port=4
  wires:
  speed_cmd/1 -> "Normalized Speed [0,1] relative to \"base freq"/1
  Gain/1 -> Estimated RPM/1
  Speed Control?/1(Out1) -> Logical Operator1/1
  Bus V/1 -> SVGEN-PWM/2(Bus Voltage)
  Enable/1 -> Logical Operator1/2
  Angle Feedback/1 -> Normalized Angle/1
  "Normalized Electrical Angle, unwrapped1"/1 -> Speed Estimator/1(In1)
  Normalize Phase [0,1]/1 -> Generate Angle vs time/2(Phase (norm))
  Generate Angle vs time/2(Reference Angle) -> Add3/2
  Normalized Angle/1 -> "Normalized Electrical Angle, unwrapped1"/1, Servo_pos_unwrap/1, Unwrapped Revolution/1, Wrap Angle/1
  Constant/1 -> Wrap Angle/2
  Add3/1 -> Wrap error2/1(In1)
  Current Controller/1(DQ V cmd) -> SVGEN-PWM/1(DQ V)
  Motor and Rotor/1(theta_rotor) -> Angle Feedback/1
  Speed Controller/2(State) -> Angle Controller/2(Initial Cond)
  Motor and Rotor/2(omega_motor) -> Servo Speed/1, Motor Efficiency/2(omega_m), Motor Emag&winding/2(Motor Speed rad/sec)
  Wrap error2/1(Out1) -> Gain9/1
  Generate Angle vs time/1(Cmd Angle (norm)) -> Angle Error/2(Commanded Rev)
  Gain9/1 -> Servo_pos/1, Actual Angle Profile/1
  Logical Operator/1 -> Speed Controller/Enable
  Speed Error/1 -> SpeedLoopRate/1
  Angle Controller/2(State) -> Unit Delay/1
  Demux/2 -> Motor Efficiency/1(I_eq), I_eq/1
  Unit Delay/1 -> Speed Controller/2(Initial Cond)
  Logical Operator1/1 -> Scope/1, Angle Controller/3(Enable1), Logical Operator/1
  Speed Estimator/1(Speed cmd) -> Gain/1, Speed Error/1
  Speed Controller/1(Out1) -> Current Loop Rate/1
  Motor Emag&winding/1(DQ current) -> Demux/1, Sample currents/1
  SpeedLoopRate/1 -> Speed Control?/1(In1), Speed Controller/1(In1)
  SVGEN-PWM/1(DQ Volts) -> Motor Emag&winding/1(DQ volts actual)
  Sample currents/1 -> Current Controller/2(DQ I feedback)
  Wrap Angle/1 -> Add3/1, Angle Error/1(Revolution)
  Servo_offset/1 -> Normalize Phase [0,1]/1
  "Normalized Speed [0,1] relative to \"base freq"/1 -> Speed Error/2, Generate Angle vs time/1(Speed)
  Current Loop Rate/1 -> Gain4/1
  Angle Error/1(Revolution Error (norm)) -> Low pass filter/1
  Low pass filter/1 -> Angle Controller/1(In1)
  "CurrentSenseMax, code right now has Controller outputting PU amps then scaled to amps going into current loop"/1 -> Current Controller/1(QI cmd), Current Cmd/1
  Gain4/1 -> Merge/1
  Merge/1 -> "CurrentSenseMax, code right now has Controller outputting PU amps then scaled to amps going into current loop"/1
  Angle Controller/1(Out1) -> Merge/2
  Motor and Rotor/3(Total Torque) -> Servo Total Torque/1
  Motor Efficiency/2(Iq) -> Motor and Rotor/1(I_Q)
  Motor Efficiency/1(Motor Efficiency) -> eta_m/1
  Load Torque/1 -> Motor and Rotor/2(Rotor Torque)

== system stackedRotor_dualEMRAX_dynInflow/Automatic Angle Commands/Enabled Subsystem ==
  In1 : Inport
  Enable : EnablePort
  Add : Sum
  Chirp : dspsrcs4/Chirp  sweep=Linear  mode=Unidirectional  f0=.1583  f1=15.83  t1=5  Tsweep=5  phase=3*pi/2  Ts=T_LOOP  spf=1  datatype=Double  OutputFrames=off
  Out1 : Outport
  wires:
  In1/1 -> Add/2
  Add/1 -> Out1/1
  Chirp/1 -> Add/1

== system stackedRotor_dualEMRAX_dynInflow/Automatic Angle Commands/Enabled Subsystem1 ==
  In1 : Inport
  Enable : EnablePort
  Out1 : Outport
  wires:
  In1/1 -> Out1/1

== system stackedRotor_dualEMRAX_dynInflow/Automatic Speed Commands/Enabled Subsystem ==
  In1 : Inport
  Enable : EnablePort
  Add : Sum
  Chirp : dspsrcs4/Chirp  sweep=Linear  mode=Unidirectional  f0=.1  f1=31  t1=4  Tsweep=4  phase=1.5*pi  Ts=T_LOOP  spf=1  datatype=Double  OutputFrames=off
  Out1 : Outport
  wires:
  In1/1 -> Add/2
  Add/1 -> Out1/1
  Chirp/1 -> Add/1

== system stackedRotor_dualEMRAX_dynInflow/Automatic Speed Commands/Enabled Subsystem1 ==
  In1 : Inport
  Enable : EnablePort
  Out1 : Outport
  wires:
  In1/1 -> Out1/1

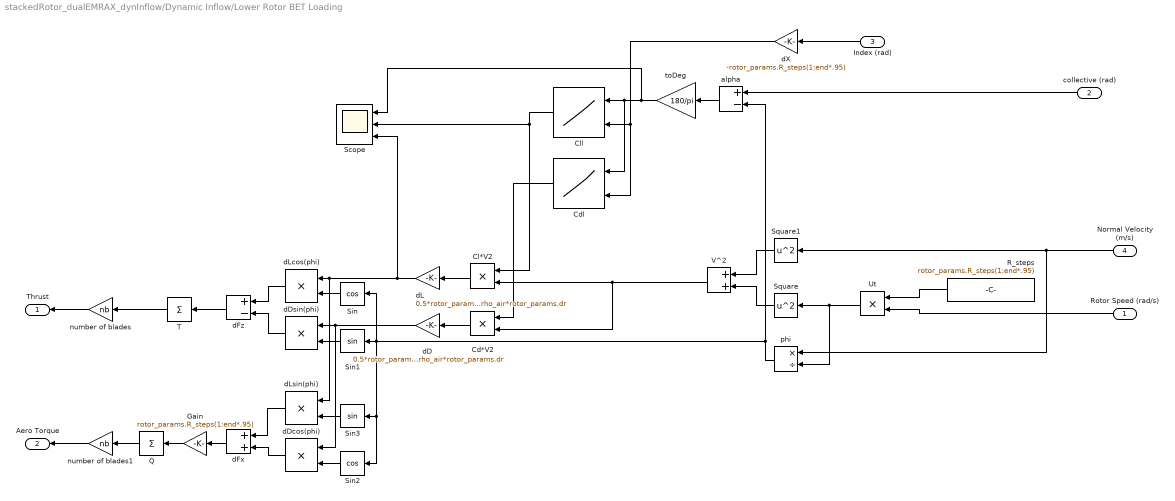
== system stackedRotor_dualEMRAX_dynInflow/Dynamic Inflow/Lower Rotor BET Loading ==
  Rotor Speed (rad/s) : Inport
  collective (rad) : Inport  Port=2
  Index (rad) : Inport  Port=3
  Normal Velocity (m/s) : Inport  Port=4
  Cd*V2 : Product
  Cdl : Lookup_n-D  BreakpointsForDimension1=AoA_sweep  BreakpointsForDimension2=x_sweep  Table=Cdl  ExtrapMethod=Clip  InternalRulePriority=Speed  RndMeth=Simplest
      settings: InputPortMap=u0,u1
  Cl*V2 : Product
  Cll : Lookup_n-D  BreakpointsForDimension1=AoA_sweep  BreakpointsForDimension2=x_sweep  Table=Cll  ExtrapMethod=Clip  InternalRulePriority=Speed  RndMeth=Simplest
      settings: InputPortMap=u0,u1
  Gain : Gain  Gain=rotor_params.R_steps(1:end*.95)
  Q : Sum  Inputs=+
  R_steps : Constant  Value=rotor_params.R_steps(1:end*.95)
  Scope : Scope  NumInputPorts=3
  Sin : Trigonometry  Operator=cos
  Sin1 : Trigonometry
  Sin2 : Trigonometry  Operator=cos
  Sin3 : Trigonometry
  Square : Math  Operator=square
  Square1 : Math  Operator=square
  T : Sum  Inputs=+
  Ut : Product
  V^2 : Sum
  alpha : Sum  Inputs=+-
  dD : Gain  Gain=0.5*rotor_params.c*rho_air*rotor_params.dr
  dDcos(phi) : Product
  dDsin(phi) : Product
  dFx : Sum
  dFz : Sum  Inputs=+-
  dL : Gain  Gain=0.5*rotor_params.c*rho_air*rotor_params.dr
  dLcos(phi) : Product
  dLsin(phi) : Product
  dX : Gain  Gain=-rotor_params.R_steps(1:end*.95)
  number of blades : Gain  Gain=nb
  number of blades1 : Gain  Gain=nb
  phi : Product  Inputs=*/
  toDeg : Gain  Gain=180/pi
  Thrust : Outport
  Aero Torque : Outport  Port=2
  wires:
  T/1 -> number of blades/1
  alpha/1 -> toDeg/1
  Normal Velocity (m/s)/1 -> phi/1, Square1/1
  Rotor Speed (rad/s)/1 -> Ut/2
  phi/1 -> Sin/1, Sin2/1, Sin3/1, Sin1/1, alpha/2
  collective (rad)/1 -> alpha/1
  Square/1 -> V^2/2
  Square1/1 -> V^2/1
  Ut/1 -> phi/2, Square/1
  V^2/1 -> Cl*V2/2, Cd*V2/2
  R_steps/1 -> Ut/1
  Cl*V2/1 -> dL/1
  Cd*V2/1 -> dD/1
  Sin/1 -> dLcos(phi)/2
  dL/1 -> Scope/3, dLsin(phi)/1, dLcos(phi)/1
  dD/1 -> dDcos(phi)/1, dDsin(phi)/1
  Sin1/1 -> dDsin(phi)/2
  dLcos(phi)/1 -> dFz/1
  dDsin(phi)/1 -> dFz/2
  dFz/1 -> T/1
  number of blades/1 -> Thrust/1
  toDeg/1 -> Scope/1, Cdl/1, Cll/1
  Cdl/1 -> Cd*V2/1
  Q/1 -> number of blades1/1
  dFx/1 -> Gain/1
  Gain/1 -> Q/1
  Cll/1 -> Cl*V2/1, Scope/2
  Index (rad)/1 -> dX/1
  dX/1 -> Cdl/2, Cll/2
  number of blades1/1 -> Aero Torque/1
  Sin2/1 -> dDcos(phi)/2
  Sin3/1 -> dLsin(phi)/2
  dDcos(phi)/1 -> dFx/2
  dLsin(phi)/1 -> dFx/1

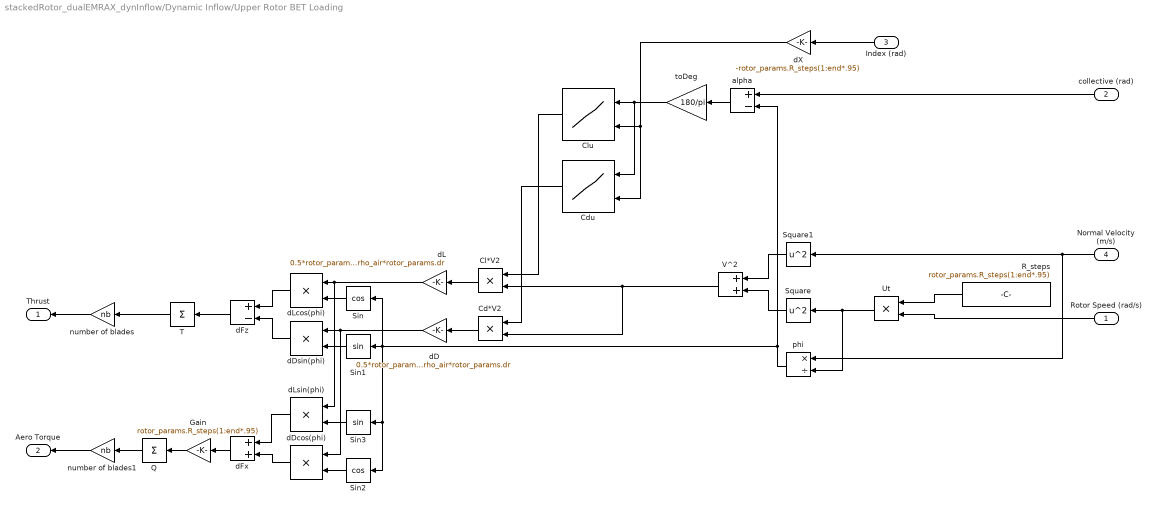
== system stackedRotor_dualEMRAX_dynInflow/Dynamic Inflow/Upper Rotor BET Loading ==
  Rotor Speed (rad/s) : Inport
  collective (rad) : Inport  Port=2
  Index (rad) : Inport  Port=3
  Normal Velocity (m/s) : Inport  Port=4
  Cd*V2 : Product
  Cdu : Lookup_n-D  BreakpointsForDimension1=AoA_sweep  BreakpointsForDimension2=x_sweep  Table=Cdu  ExtrapMethod=Clip  InternalRulePriority=Speed  RndMeth=Simplest
      settings: InputPortMap=u0,u1
  Cl*V2 : Product
  Clu : Lookup_n-D  BreakpointsForDimension1=AoA_sweep  BreakpointsForDimension2=x_sweep  Table=Clu  ExtrapMethod=Clip  InternalRulePriority=Speed  RndMeth=Simplest
      settings: InputPortMap=u0,u1
  Gain : Gain  Gain=rotor_params.R_steps(1:end*.95)
  Q : Sum  Inputs=+
  R_steps : Constant  Value=rotor_params.R_steps(1:end*.95)
  Sin : Trigonometry  Operator=cos
  Sin1 : Trigonometry
  Sin2 : Trigonometry  Operator=cos
  Sin3 : Trigonometry
  Square : Math  Operator=square
  Square1 : Math  Operator=square
  T : Sum  Inputs=+
  Ut : Product
  V^2 : Sum
  alpha : Sum  Inputs=+-
  dD : Gain  Gain=0.5*rotor_params.c*rho_air*rotor_params.dr
  dDcos(phi) : Product
  dDsin(phi) : Product
  dFx : Sum
  dFz : Sum  Inputs=+-
  dL : Gain  Gain=0.5*rotor_params.c*rho_air*rotor_params.dr
  dLcos(phi) : Product
  dLsin(phi) : Product
  dX : Gain  Gain=-rotor_params.R_steps(1:end*.95)
  number of blades : Gain  Gain=nb
  number of blades1 : Gain  Gain=nb
  phi : Product  Inputs=*/
  toDeg : Gain  Gain=180/pi
  Thrust : Outport
  Aero Torque : Outport  Port=2
  wires:
  T/1 -> number of blades/1
  alpha/1 -> toDeg/1
  Normal Velocity (m/s)/1 -> phi/1, Square1/1
  Rotor Speed (rad/s)/1 -> Ut/2
  phi/1 -> Sin/1, Sin2/1, Sin3/1, Sin1/1, alpha/2
  collective (rad)/1 -> alpha/1
  Square/1 -> V^2/2
  Square1/1 -> V^2/1
  Ut/1 -> phi/2, Square/1
  V^2/1 -> Cl*V2/2, Cd*V2/2
  R_steps/1 -> Ut/1
  Cl*V2/1 -> dL/1
  Cd*V2/1 -> dD/1
  Sin/1 -> dLcos(phi)/2
  dL/1 -> dLsin(phi)/1, dLcos(phi)/1
  dD/1 -> dDcos(phi)/1, dDsin(phi)/1
  Sin1/1 -> dDsin(phi)/2
  dLcos(phi)/1 -> dFz/1
  dDsin(phi)/1 -> dFz/2
  dFz/1 -> T/1
  number of blades/1 -> Thrust/1
  toDeg/1 -> Cdu/1, Clu/1
  Cdu/1 -> Cd*V2/1
  Q/1 -> number of blades1/1
  dFx/1 -> Gain/1
  Gain/1 -> Q/1
  Clu/1 -> Cl*V2/1
  Index (rad)/1 -> dX/1
  dX/1 -> Cdu/2, Clu/2
  number of blades1/1 -> Aero Torque/1
  Sin2/1 -> dDcos(phi)/2
  Sin3/1 -> dLsin(phi)/2
  dDcos(phi)/1 -> dFx/2
  dLsin(phi)/1 -> dFx/1

== system stackedRotor_dualEMRAX_dynInflow/Find Index Angle/If Action Subsystem ==
  In1 : Inport
  Action Port : ActionPort  ActionPortLabel=if(u1 >= 0)
  Constant : Constant
  Mod : Math  Operator=mod
  Out1 : Outport
  wires:
  Constant/1 -> Mod/2
  In1/1 -> Mod/1
  Mod/1 -> Out1/1

== system stackedRotor_dualEMRAX_dynInflow/Find Index Angle/If Action Subsystem1 ==
  In1 : Inport
  Action Port : ActionPort  ActionPortLabel=else
  Constant : Constant
  Gain : Gain  Gain=-1
  Mod : Math  Operator=rem
  Out1 : Outport
  wires:
  Constant/1 -> Mod/2
  In1/1 -> Mod/1
  Mod/1 -> Gain/1
  Gain/1 -> Out1/1

== system stackedRotor_dualEMRAX_dynInflow/Find Index Angle/If Action Subsystem2 ==
  In1 : Inport
  Action Port : ActionPort  ActionPortLabel="if(.25 < u1  & u1 <= .75)"
  Constant : Constant  Value=.5
  Subtract : Sum  Inputs=+-
  Out1 : Outport
  wires:
  Constant/1 -> Subtract/2
  In1/1 -> Subtract/1
  Subtract/1 -> Out1/1

== system stackedRotor_dualEMRAX_dynInflow/Find Index Angle/If Action Subsystem3 ==
  In1 : Inport
  Action Port : ActionPort  ActionPortLabel=elseif(u1 > .75)
  Constant : Constant
  Subtract : Sum  Inputs=+-
  Out1 : Outport
  wires:
  Constant/1 -> Subtract/2
  In1/1 -> Subtract/1
  Subtract/1 -> Out1/1

== system stackedRotor_dualEMRAX_dynInflow/Find Index Angle/If Action Subsystem4 ==
  In1 : Inport
  Action Port : ActionPort  ActionPortLabel=else
  Out1 : Outport
  wires:
  In1/1 -> Out1/1

== system stackedRotor_dualEMRAX_dynInflow/Follower/Angle Controller ==
  In1 : Inport
  Initial Cond : Inport  Port=2
  Enable1 : Inport  Port=3
  Angle Controller DT_PID saturate P : Subsystem
  Max error : Saturate  UpperLimit=PID_pos_error_sat  LowerLimit=-PID_pos_error_sat
  Out1 : Outport  InitialOutput=[0]
  State : Outport  Port=2  InitialOutput=[0]
  wires:
  Initial Cond/1 -> Angle Controller DT_PID saturate P/2(Iniitial Cond)
  Enable1/1 -> Angle Controller DT_PID saturate P/Enable
  Angle Controller DT_PID saturate P/1(Out1) -> Out1/1
  Angle Controller DT_PID saturate P/2(Integrator) -> State/1
  In1/1 -> Max error/1
  Max error/1 -> Angle Controller DT_PID saturate P/1(In1)

== system stackedRotor_dualEMRAX_dynInflow/Follower/Angle Error ==
  Revolution : Inport
  Commanded Rev : Inport  Port=2
  Add4 : Sum  Inputs=-+
  Angle Error Calc Deg : Scope
  Gain2 : Gain  Gain=360
  To Workspace3 : ToWorkspace  VariableName=Angle_err_follower  SaveFormat=Timeseries  SampleTime=-1
  Wrap error : Subsystem
  Revolution Error (norm) : Outport
  tag scope: angle_err_follwer=global
  wires:
  Revolution/1 -> Add4/1
  Wrap error/1(Out1) -> [angle_err_follwer], Revolution Error (norm)/1, Gain2/1
  Gain2/1 -> To Workspace3/1, Angle Error Calc Deg/1
  Add4/1 -> Wrap error/1(In1)
  Commanded Rev/1 -> Add4/2

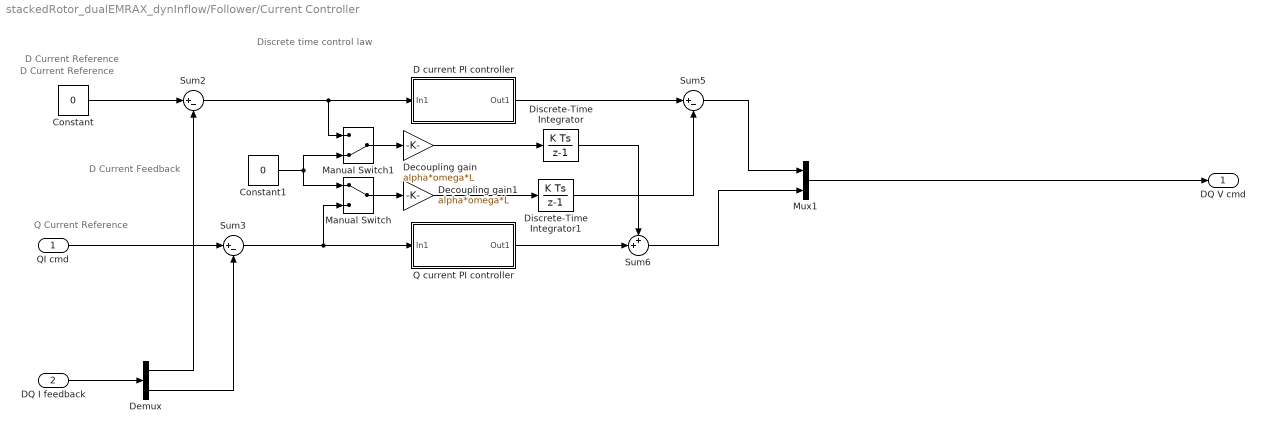
== system stackedRotor_dualEMRAX_dynInflow/Follower/Current Controller ==
  note: D Current Reference
  note: D Current Feedback
  note: D Current Reference
  note: Q Current Reference
  note: Discrete
      | time control
      | law
  QI cmd : Inport
  DQ I feedback : Inport  Port=2
  Constant : Constant  Value=0
  Constant1 : Constant  Value=0
  D current PI controller : Subsystem
  Decoupling gain : Gain  Gain=alpha*omega*L
  Decoupling gain1 : Gain  Gain=alpha*omega*L
  Demux : Demux  Outputs=2
  Discrete-Time Integrator : DiscreteIntegrator  SampleTime=T_LOOP  ICPrevOutput=DiscIntNeverNeededParam  ICPrevScaledInput=DiscIntNeverNeededParam
  Discrete-Time Integrator1 : DiscreteIntegrator  SampleTime=T_LOOP  ICPrevOutput=DiscIntNeverNeededParam  ICPrevScaledInput=DiscIntNeverNeededParam
  Manual Switch : ManualSwitch
  Manual Switch1 : ManualSwitch  CurrentSetting=0
  Mux1 : Mux  Inputs=2
  Q current PI controller : Subsystem
  Sum2 : Sum  Inputs=|+-
  Sum3 : Sum  Inputs=|+-
  Sum5 : Sum  Inputs=|+-
  Sum6 : Sum  Inputs=++|
  DQ V cmd : Outport
  wires:
  Mux1/1 -> DQ V cmd/1
  Sum2/1 -> D current PI controller/1(In1), Manual Switch1/1
  Sum3/1 -> Q current PI controller/1(In1), Manual Switch/2
  Constant/1 -> Sum2/1
  D current PI controller/1(Out1) -> Sum5/1
  Q current PI controller/1(Out1) -> Sum6/2
  Discrete-Time Integrator/1 -> Sum6/1
  Discrete-Time Integrator1/1 -> Sum5/2
  QI cmd/1 -> Sum3/1
  Decoupling gain1/1 -> Discrete-Time Integrator1/1
  Decoupling gain/1 -> Discrete-Time Integrator/1
  Manual Switch/1 -> Decoupling gain1/1
  Manual Switch1/1 -> Decoupling gain/1
  Constant1/1 -> Manual Switch1/2, Manual Switch/1
  Sum5/1 -> Mux1/1
  Sum6/1 -> Mux1/2
  DQ I feedback/1 -> Demux/1
  Demux/1 -> Sum2/2
  Demux/2 -> Sum3/2

== system stackedRotor_dualEMRAX_dynInflow/Follower/Generate Angle vs time ==
  Speed : Inport
  Phase (norm) : Inport  Port=2
  Add5 : Sum
  Constant1 : Constant
  Constant3 : Constant
  Discrete-Time Integrator : DiscreteIntegrator  SampleTime=-1  ICPrevOutput=DiscIntNeverNeededParam  ICPrevScaledInput=DiscIntNeverNeededParam
  Normalized Mech Angle : Gain  Gain=BASE_FREQ/(POLES/2)
  Wrap command : Math  Operator=mod  SignedPower=on
  Wrap command1 : Math  Operator=mod  SignedPower=on
  Cmd Angle (norm) : Outport
  Reference Angle : Outport  Port=2
  wires:
  Constant1/1 -> Wrap command/2
  Discrete-Time Integrator/1 -> Normalized Mech Angle/1
  Add5/1 -> Wrap command/1
  Speed/1 -> Discrete-Time Integrator/1
  Phase (norm)/1 -> Add5/1
  Wrap command/1 -> Cmd Angle (norm)/1
  Constant3/1 -> Wrap command1/2
  Normalized Mech Angle/1 -> Wrap command1/1, Add5/2
  Wrap command1/1 -> Reference Angle/1

== system stackedRotor_dualEMRAX_dynInflow/Follower/Motor Emag&winding ==
  note: Winding model
  DQ volts actual : Inport
  Motor Speed rad/sec : Inport  Port=2
  D Q currents : Scope
  Demux1 : Demux  Outputs=2
  Motor Back EMF : Gain  Gain=Ke_motor/sqrt(3)
  Mux2 : Mux  Inputs=2
  Subsystem : Subsystem
  Sum4 : Sum  Inputs=|+-
  DQ current : Outport
  wires:
  Motor Speed rad/sec/1 -> Motor Back EMF/1, Subsystem/2(Motor speed rad/sec)
  Mux2/1 -> Subsystem/1(DQ voltages)
  Demux1/1 -> Mux2/1
  Demux1/2 -> Sum4/1
  Sum4/1 -> Mux2/2
  Motor Back EMF/1 -> Sum4/2
  DQ volts actual/1 -> Demux1/1
  Subsystem/1(DQ currents) -> DQ current/1, D Q currents/1

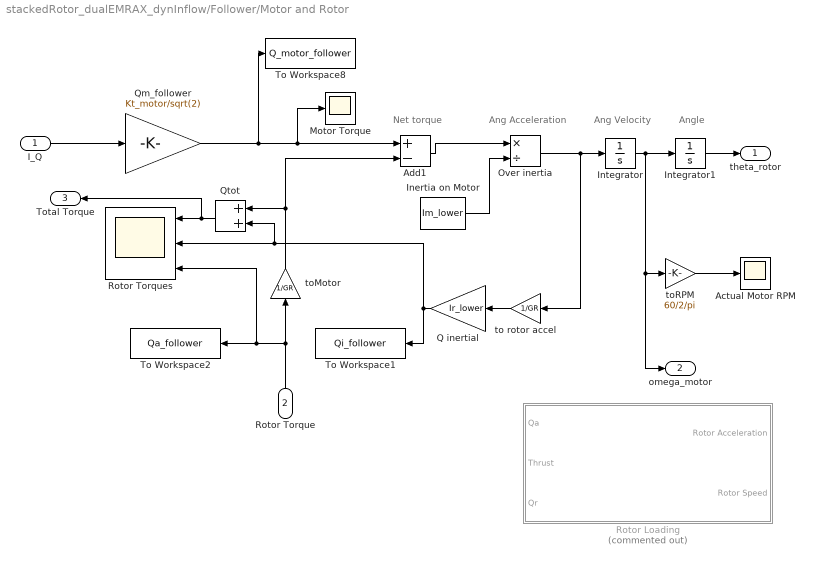
== system stackedRotor_dualEMRAX_dynInflow/Follower/Motor and Rotor ==
  note: Ang Acceleration
  note: Angle
  note: Ang Velocity
  note: Net torque
  I_Q : Inport
  Rotor Torque : Inport  Port=2
  Actual Motor RPM : Scope
  Add1 : Sum  Inputs=+-
  "Inertia on Motor " : Constant  Value=Im_lower
  Integrator : Integrator  InitialCondition=InitialRPM*2*pi/60
  Integrator1 : Integrator
  Motor Torque : Scope
  Over inertia : Product  Inputs=*/
  Q inertial : Gain  Gain=Ir_lower
  Qm_follower : Gain  Gain=Kt_motor/sqrt(2)
  Qtot : Sum
  Rotor Loading : Subsystem  Commented=on
  Rotor Torques : Scope  NumInputPorts=3
  To Workspace1 : ToWorkspace  VariableName=Qi_follower  SaveFormat=Timeseries  SampleTime=-1
  To Workspace2 : ToWorkspace  VariableName=Qa_follower  SaveFormat=Timeseries  SampleTime=-1
  To Workspace8 : ToWorkspace  VariableName=Q_motor_follower  SaveFormat=Timeseries  SampleTime=-1
  to rotor accel : Gain  Gain=1/GR
  toMotor : Gain  Gain=1/GR
  toRPM : Gain  Gain=60/2/pi
  theta_rotor : Outport
  omega_motor : Outport  Port=2
  Total Torque : Outport  Port=3
  wires:
  Integrator/1 -> Integrator1/1, omega_motor/1, toRPM/1
  I_Q/1 -> Qm_follower/1
  Over inertia/1 -> to rotor accel/1, Integrator/1
  Integrator1/1 -> theta_rotor/1
  Add1/1 -> Over inertia/1
  toRPM/1 -> Actual Motor RPM/1
  to rotor accel/1 -> Q inertial/1
  "Inertia on Motor "/1 -> Over inertia/2
  Qm_follower/1 -> To Workspace8/1, Motor Torque/1, Add1/1
  Rotor Torque/1 -> To Workspace2/1, Rotor Torques/3, toMotor/1
  Q inertial/1 -> To Workspace1/1, Rotor Torques/2, Qtot/2
  toMotor/1 -> Qtot/1, Add1/2
  Qtot/1 -> Rotor Torques/1, Total Torque/1
